simulink model "calc_coeff"  (R2020b)
settings: Solver=FixedStepDiscrete  StartTime=0.0  StopTime=stopTime  FixedStep=2.0833333333333333e-05  RelTol=1e-3
values from neighbouring files (symbols this model uses):
  fs_bilinear = 2*pi*cf/tan(2*pi*cf*tdres/2)    [modelparameters.m]
settings Model: Creator=Ross  LastModifiedBy=conno
settings DataIOCC: SaveOutput=off  SaveTime=off  ReturnWorkspaceOutputs=off
settings OptimizationCC: BlockReduction=off  ConditionallyExecuteInputs=off  DefaultParameterBehavior=Inlined
settings DebuggingCC: ReadBeforeWriteMsg=DisableAll  WriteAfterWriteMsg=DisableAll  WriteAfterReadMsg=DisableAll  AlgebraicLoopMsg=error  MultiTaskDSMMsg=none  SingleTaskRateTransMsg=error  PregeneratedLibrarySubsystemCodeDiagnostic=none  ArithmeticOperatorsInVariantConditions=warning
settings HardwareCC: ProdBitPerPointer=32  ProdBitPerSizeT=32  ProdBitPerPtrDiffT=32  ProdLargestAtomicFloat=None  ProdIntDivRoundTo=Undefined  ProdEndianess=Unspecified  ProdWordSize=32  ProdHWDeviceType=ASIC/FPGA->ASIC/FPGA  TargetBitPerPointer=64  TargetBitPerSizeT=64  TargetBitPerPtrDiffT=64  TargetLongLongMode=on  TargetIntDivRoundTo=Zero  TargetEndianess=LittleEndian  TargetWordSize=64  TargetHWDeviceType=Custom Processor->MATLAB Host Computer  ProdEqTarget=off
settings ModelReferenceCC: UpdateModelReferenceTargets=IfOutOfDate
settings SFSimCC: SFSimEcho=off  SimUseLocalCustomCode=off  CustomCodeUndefinedFunction=UseInterfaceOnly
settings RTWCC: RTWUseLocalCustomCode=off

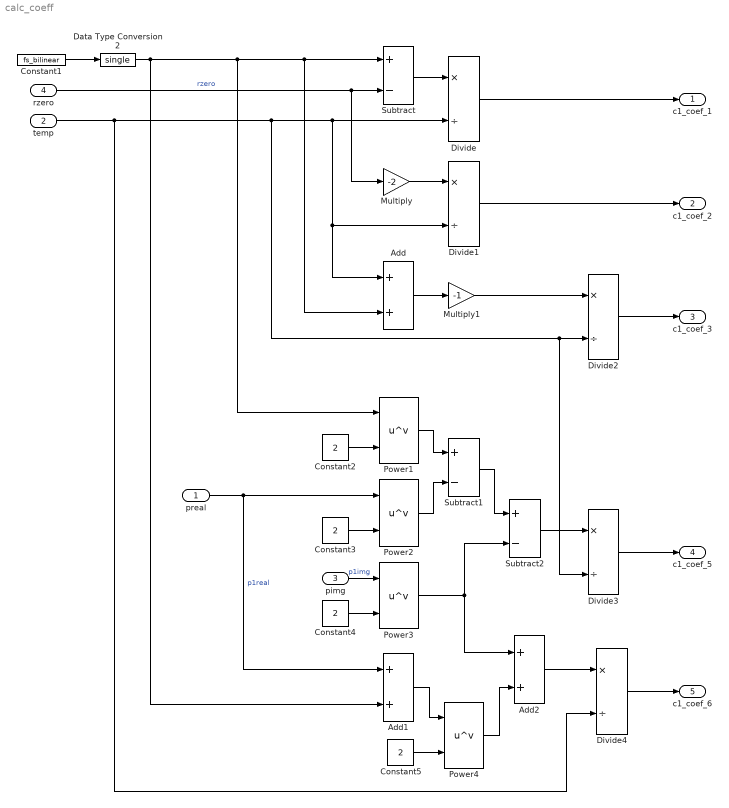
== system calc_coeff ==
  preal : Inport  OutDataTypeStr=single  PortDimensions=1  SampleTime=[2.0833333333333333e-05,0]
  temp : Inport  Port=2  OutDataTypeStr=single  PortDimensions=1  SampleTime=[2.0833333333333333e-05,0]
  pimg : Inport  Port=3  OutDataTypeStr=single  PortDimensions=1
  rzero : Inport  Port=4  OutDataTypeStr=single  PortDimensions=1  SampleTime=[2.0833333333333333e-05,0]
  Add : Sum
  Add1 : Sum
  Add2 : Sum
  Constant1 : Constant  Value=fs_bilinear  SampleTime=-1
  Constant{2..5} (4 alike) : Constant  Value=2  OutDataTypeStr=Inherit: Inherit via back propagation  SampleTime=-1
  Data Type Conversion2 : DataTypeConversion  OutDataTypeStr=single  RndMeth=Nearest
  Divide{,1..4} (5 alike) : Product  Inputs=*/
  Multiply : Gain  Gain=-2
  Multiply1 : Gain  Gain=-1
  Power{1..4} (4 alike) : Math  Operator=pow  SaturateOnIntegerOverflow=on
  Subtract : Sum  Inputs=+-
  Subtract1 : Sum  Inputs=+-
  Subtract2 : Sum  Inputs=+-
  c1_coef_1 : Outport  OutDataTypeStr=single  PortDimensions=1  SampleTime=[2.0833333333333333e-05,0]
  c1_coef_2 : Outport  Port=2  OutDataTypeStr=single  PortDimensions=1  SampleTime=[2.0833333333333333e-05,0]
  c1_coef_3 : Outport  Port=3  OutDataTypeStr=single  PortDimensions=1  SampleTime=[2.0833333333333333e-05,0]
  c1_coef_5 : Outport  Port=4  OutDataTypeStr=single  PortDimensions=1  SampleTime=[2.0833333333333333e-05,0]
  c1_coef_6 : Outport  Port=5  OutDataTypeStr=single  PortDimensions=1  SampleTime=[2.0833333333333333e-05,0]
  wires:
  Constant1/1 -> Data Type Conversion2/1
  rzero/1 -> Subtract/2, Multiply/1  "rzero"
  Data Type Conversion2/1 -> Subtract/1, Add/2, Power1/1, Add1/2
  temp/1 -> Divide2/2, Divide3/2, Divide/2, Divide1/2, Add/1, Divide4/2
  Subtract/1 -> Divide/1
  Divide/1 -> c1_coef_1/1
  Multiply/1 -> Divide1/1
  Divide1/1 -> c1_coef_2/1
  Add/1 -> Multiply1/1
  Multiply1/1 -> Divide2/1
  Divide2/1 -> c1_coef_3/1
  Constant2/1 -> Power1/2
  Power1/1 -> Subtract1/1
  Power2/1 -> Subtract1/2
  Constant3/1 -> Power2/2
  preal/1 -> Power2/1, Add1/1  "p1real"
  Constant4/1 -> Power3/2
  pimg/1 -> Power3/1  "p1img"
  Power3/1 -> Add2/1, Subtract2/2
  Subtract1/1 -> Subtract2/1
  Subtract2/1 -> Divide3/1
  Divide3/1 -> c1_coef_5/1
  Constant5/1 -> Power4/2
  Add1/1 -> Power4/1
  Power4/1 -> Add2/2
  Add2/1 -> Divide4/1
  Divide4/1 -> c1_coef_6/1
